simulink model "Galvo_sys_Cdisc_Pcont_cc_v64_proto_v13"  (R2013a)
settings: Solver=ode45  StartTime=0.0  StopTime=25e-3  FixedStep=FS  MaxStep=1e-5  RelTol=1e-3  AbsTol=1e-5
PreLoadFcn:
  | vname=@(x) inputname(1);
  | paramCtrl=evalin('base','paramCtrl;');
  | I_LIM=str2num(paramCtrl.I_LIM);
  | Kbc=str2num(paramCtrl.Kbc);
  | FS=evalin('base','FS;');
InitFcn:
  | %%%%%%  set scope time range
  | T_STOP=str2num(get_param(gcs,'StopTime'));
  | if numel(T_STOP) > 1
  |    T_STOP=T_STOP(2);
  | else
  |    T_STOP=T_STOP(1);
  | end
  | T_STOP=num2str(T_STOP);
  | 
  | %%%%%%  set scope time range in system @init_callback_fct
  | T_STOP=num2str(str2num(get_param(gcs,'StopTime')));
  | 
  | childs = allchild(0);
  | sol=strfind(upper(get(allchild(0),'Tag')),'VIEWER_PARAMETERS');
  | 
  | if iscell(sol)
  |    ind=find(~cellfun(@isempty, strfind(upper(get(allchild(0),'Tag')),'VIEWER_PARAMETERS')));
  | else
  |    ind=sol;
  | end
  | %ind=find(~cellfun(@isempty, {strfind(upper(get(allchild(0),'Tag')),'VIEWER_PARAMETERS'),[]}))
  | if ~isempty(ind)
  |    for k=1:length(childs(ind))
  |       set_param(getfield(get(childs(ind(k)),'UserData'),'block'),'TimeRange',T_STOP);
  |       get_param(getfield(get(childs(ind(k)),'UserData'),'block'),'TimeRange');
  | %    set_param(getfield(get(childs(ind),'UserData'),'block'),'TimeRange',T_STOP);
  | %    get_param(getfield(get(childs(ind),'UserData'),'block'),'TimeRange');
  |    end
  | else
  |     warning(sprintf('VIEWER_PARAMETERS object not found\nOpen the config dialog by hand for the first sim start'))
  | end
StartFcn:
  | I_LIM=str2num(paramCtrl.I_LIM);
  | Kbc=str2num(paramCtrl.Kbc);
  | %FS=evalin('base','FS;');
values from neighbouring files (symbols this model uses):
  Lc = 170e-6    (= 0.00017)    [GalvoModel_v6_sys.m]    (also in Galvo_process_analyze.m)
  Rc = 1.5    [GalvoModel_v6_sys.m]    (also in Galvo_process_analyze.m; frequenzgang_nichtinvert_opamp_koblitz_eas.m = 1)
  Rsh = 0.003    [GalvoModel_v6_sys.m]    (also in Galvo_sys_proto_v13_OFFSETS_MODEL_PT1B_proc.m = 0.075; frequenzgang_nichtinvert_opamp_koblitz_eas.m = 0.015)
undefined symbols (not defined in the file or in its folder): JR, KBM, KFR, KMT, KPOS1, KshM, KTB
libraries: simulink x4, simulink_extras x1, dspsigops x1
settings Model: BufferReuse=off  Creator=mainster  LastModifiedBy=mainster
settings SolverCC: AutoInsertRateTranBlk=on
settings DataIOCC: LimitDataPoints=off  SaveOutput=off  SaveTime=off
settings OptimizationCC: BlockReduction=off  InlineParams=on  OptimizeBlockIOStorage=off  BufferReuse=off  ExpressionFolding=off  LocalBlockOutputs=off
settings DebuggingCC: ArtificialAlgebraicLoopMsg=none  InitInArrayFormatMsg=none
settings HardwareCC: ProdLargestAtomicInteger=Long  ProdLargestAtomicFloat=Double  ProdEndianess=LittleEndian  ProdHWDeviceType=ARM Compatible->ARM Cortex
settings ModelReferenceCC: ModelReferenceNumInstancesAllowed=Single

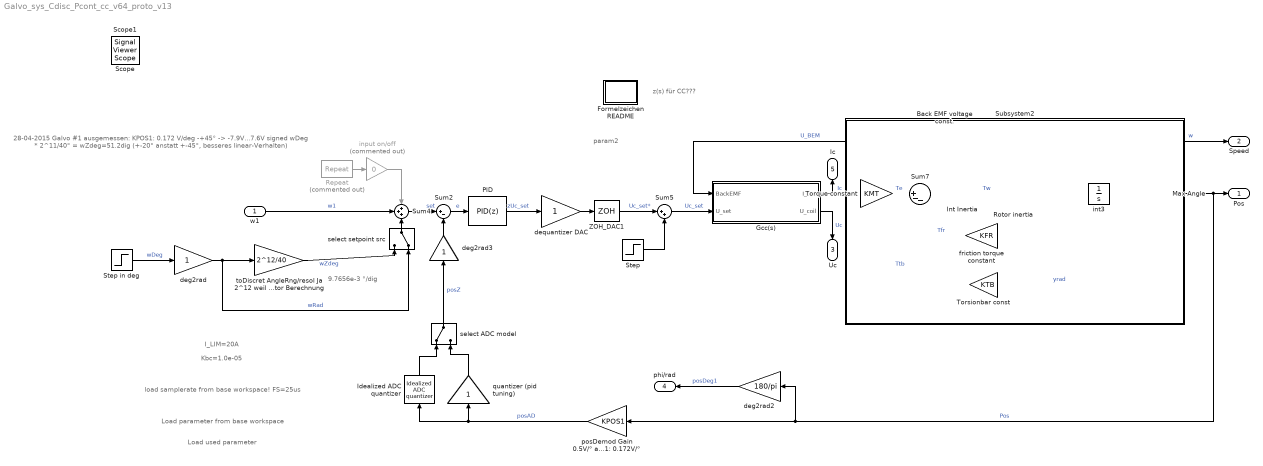
== system Galvo_sys_Cdisc_Pcont_cc_v64_proto_v13 ==
  note: 9.7656e-3 °/dig
  note: 28-04-2015
      | Galvo #1 ausgemessen:
      |
      | KPOS1: 0.172 V/deg
      |  -+45° ->  -7.9V...7.6V
      |
      | signed wDeg * 2^11/40° = wZdeg=51.2dig
      | (+-20° anstatt +-45°, besseres
      | linear-Verhalten)
  note: z(s) für
      | CC???
  note: param2
  note: I_LIM=20A
  note: Kbc=1.0e-05
  note: load samplerate from
      | base workspace!
      | FS=25us
  note: Load parameter from
      | base workspace
  note: Load used parameter
  w1 : Inport
  Back EMF voltage const. : Gain  Gain=KBM
  Formelzeichen README : Subsystem
  Gcc(s) : Subsystem
      mask Display:
      | %str=sprintf('%s',get(gcbh,'ModelName'));
      | port_label('input', 2, 'I/U_{Set}','texmode','on')
      | color('red');
      | port_label('input', 1, 'U_{BEM}','texmode','on')
      | color('black');
      | port_label('output', 1, 'I_{Coil}','texmode','on')
      | port_label('output', 2, 'U_{Coil}','texmode','on')
      | %text(.05,.98,['{\fontsize{12}\it\bf' strrep(str,'_',' ') '}'],'horizontalAlignment','left','verticalAlignment','top','texmode','on')
      | text(.5,0.95,['{\fontsize{12}\it\bfG_{cc}(s)}'],'horizontalAlignment','center','verticalAlignment','top','texmode','on')
      | %text(.5,0.45,['{\fontsize{8}\itKpcc=' num2str(get_param([gcb '/Cc(s)'],'P')) '}'],'horizontalAlignment','center','verticalAlignment','top','texmode','on')
      | %text(.5,0.25,['{\fontsize{8}\itKshM=' num2str(evalin('base',get_param([gcb '/shuntMonGain'],'Gain'))) '}'],'horizontalAlignment','center','verticalAlignment','top','texmode','on')
      | 
      | %text(.15,.05,['{\fontsize{10}\itmechanics}'],'horizontalAlignment','left','verticalAlignment','bottom','texmode','on')
  Idealized ADC quantizer : simulink_extras/Additional Discrete/Idealized ADC quantizer  NumberOfConverterBits=12  Vmin=-1.25  Vmax=1.25  OutputDataType=int16  OutputNegativeValues=on
  Int Inertia : Integrator
  Max Angle : Saturate  UpperLimit=20*pi/180*1e3  LowerLimit=-20*pi/180*1e3
      settings: AttributesFormatString=Max=%<UpperLimit>\nMin=%<LowerLimit>
  PID : simulink/Continuous/PID Controller  Controller=PID  TimeDomain=Discrete-time  SampleTime=FS  IntegratorMethod=Forward Euler  FilterMethod=Forward Euler  Form=Parallel  P=133.868463594608  I=12873.0781764522  D=0.158359314809688  N=29290.0509767599  InitialConditionSource=internal  InitialConditionForIntegrator=0  InitialConditionForFilter=0  ExternalReset=none  IgnoreLimit=on  LimitOutput=on  UpperSaturationLimit=2047  LowerSaturationLimit=-2048  LinearizeAsGain=off  AntiWindupMode=clamping  Kb=0.1  TrackingMode=off  Kt=0  PParamMin=[]  PParamMax=[]  IParamMin=[]  IParamMax=[]  DParamMin=[]  DParamMax=[]  NParamMin=[]  NParamMax=[]  KbParamMin=[]  KbParamMax=[]  KtParamMin=[]  KtParamMax=[]  POutMin=[]  POutMax=[]  IOutMin=[]  IOutMax=[]  DOutMin=[]  DOutMax=[]  NOutMin=[]  NOutMax=[]  KbOutMin=[]  KbOutMax=[]  KtOutMin=[]  KtOutMax=[]  IntegratorOutMin=[]  IntegratorOutMax=[]  FilterOutMin=[]  FilterOutMax=[]  SumOutMin=[]  SumOutMax=[]  SumI1OutMin=[]  SumI1OutMax=[]  SumI2OutMin=[]  SumI2OutMax=[]  SumI3OutMin=[]  SumI3OutMax=[]  SumDOutMin=[]  SumDOutMax=[]  SaturationOutMin=[]  SaturationOutMax=[]  IntegratorContinuousStateAttributes=''  IntegratorStateMustResolveToSignalObject=off  IntegratorRTWStateStorageClass=Auto  FilterContinuousStateAttributes=''  FilterStateMustResolveToSignalObject=off  FilterRTWStateStorageClass=Auto
      settings: AttributesFormatString=Kp: %<P>\nKi: %<I>\nKd: %<D>\nuplim: %<UpperSaturationLimit>\nlolim: %<LowerSaturationLimit>
  Repeat : dspsigops/Repeat  Commented=on  N=length(str2num(get_param([gcs '/Sequence Stair'], 'OutValues')))  InputProcessing=Columns as channels (frame based)  RateOptions=Allow multirate processing  ic=0  mode=Unused parameter value
  Rotor inertia : Gain  Gain=1/JR
  Step : Step  Time=100e-3  After=0  SampleTime=0
      settings: AttributesFormatString=Ampl.: %<After>\ntime:%<Time>
  Step in deg : Step  Time=1e-3  SampleTime=0  ZeroCross=off
      settings: AttributesFormatString=Ampl.: %<After>\ntime:%<Time>
  Subsystem2 : Subsystem
      mask Display: text(.05,.05,['{\fontsize{13}\it\bfGalvo mechanic}'],'horizontalAlignment','left','verticalAlignment','bottom','texmode','on')
  Sum2 : Sum  Inputs=|+-
  Sum4 : Sum  Inputs=+++
  Sum5 : Sum  Inputs=|++
  Sum7 : Sum  Inputs=||+--
  Torque constant : Gain  Gain=KMT
  Torsionbar const : Gain  Gain=KTB
  ZOH_DAC1 : ZeroOrderHold  SampleTime=FS
  deg2rad : Gain
  deg2rad2 : Gain  Gain=180/pi
  deg2rad3 : Gain
  dequantizer DAC : Gain
  friction torque constant : Gain  Gain=KFR
  input on/off : Gain  Commented=on  Gain=0  SampleTime=FS
  int3 : Integrator
  "posDemod Gain 0.5V/° ausgemessen bei Galvo #1: 0.172V/° " : Gain  Gain=KPOS1
  quantizer (pid tuning) : Gain
  select ADC model : ManualSwitch
  select setpoint src : ManualSwitch  CurrentSetting=0
  "toDiscret AngleRng/resol Ja 2^12 weil nur Faktor Berechnung " : Gain  Gain=2^12/40
  Pos : Outport
  Speed : Outport  Port=2
  Uc : Outport  Port=3
  phi/rad : Outport  Port=4
  Ic : Outport  Port=5
  Scope : SignalViewerScope  IOType=viewer  NumInputPorts=5  RefreshTime=0.033391
      settings: ShowLegends=on  TimeRange=0.025  YMin=0~-500~0~0~-500  YMax=8~2500~8~400~2500
  Scope1 : SignalViewerScope  IOType=viewer  NumInputPorts=5  RefreshTime=0.035000
      settings: ShowLegends=on  TimeRange=0.025  YMin=-10~0~-0.5~-20~0  YMax=10~1.5~1~30~120
  wires:
  w1/1 -> Sum4/2  "w1"
  Repeat/1 -> input on/off/1
  Sum2/1 -> PID/1  "e"
  Sum4/1 -> Sum2/1  "set"
  Step in deg/1 -> deg2rad/1  "wDeg"
  input on/off/1 -> Sum4/1
  Step/1 -> Sum5/2
  int3/1 -> Max Angle/1, Torsionbar const/1  "yrad"
  Int Inertia/1 -> Rotor inertia/1  "Tw"
  Sum7/1 -> Int Inertia/1
  Rotor inertia/1 -> Speed/1, int3/1, Back EMF voltage const./1, friction torque constant/1  "w"
  friction torque constant/1 -> Sum7/3  "Tfr"
  Max Angle/1 -> deg2rad2/1, "posDemod Gain 0.5V/° ausgemessen bei Galvo #1: 0.172V/° "/1, Pos/1  "Pos"
  Torque constant/1 -> Sum7/1  "Te"
  Torsionbar const/1 -> Sum7/2  "Ttb"
  PID/1 -> dequantizer DAC/1  "zUc_set"
  Sum5/1 -> Gcc(s)/2(U_set)  "Uc_set"
  Gcc(s)/1(I_coil) -> Torque constant/1, Ic/1  "Ic"
  Gcc(s)/2(U_coil) -> Uc/1  "Uc"
  "posDemod Gain 0.5V/° ausgemessen bei Galvo #1: 0.172V/° "/1 -> Idealized ADC quantizer/1, quantizer (pid tuning)/1  "posAD"
  deg2rad2/1 -> phi/rad/1  "posDeg1"
  Back EMF voltage const./1 -> Gcc(s)/1(BackEMF)  "U_BEM"
  ZOH_DAC1/1 -> Sum5/1  "Uc_set*"
  Idealized ADC quantizer/1 -> select ADC model/1
  select ADC model/1 -> deg2rad3/1  "posZ"
  "toDiscret AngleRng/resol Ja 2^12 weil nur Faktor Berechnung "/1 -> select setpoint src/1  "wZdeg"
  select setpoint src/1 -> Sum4/3
  deg2rad3/1 -> Sum2/2
  deg2rad/1 -> select setpoint src/2, "toDiscret AngleRng/resol Ja 2^12 weil nur Faktor Berechnung "/1  "wRad"
  quantizer (pid tuning)/1 -> select ADC model/2
  dequantizer DAC/1 -> ZOH_DAC1/1

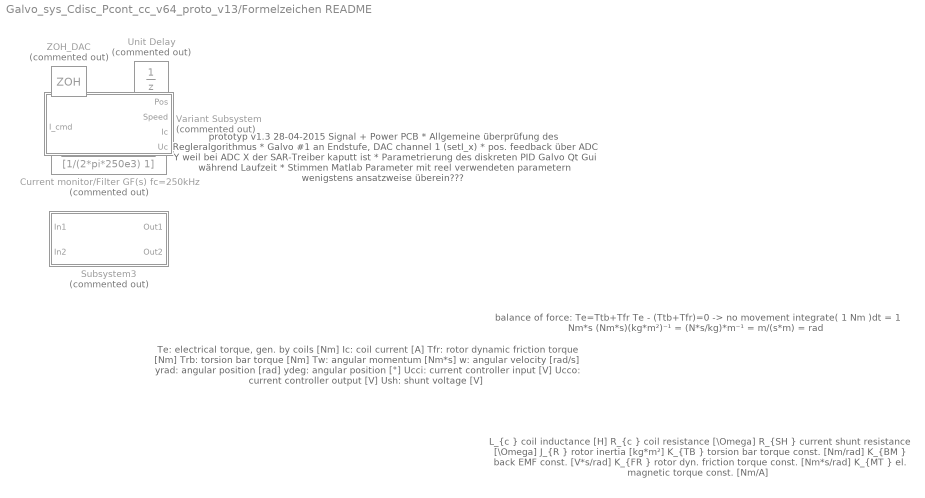
== system Galvo_sys_Cdisc_Pcont_cc_v64_proto_v13/Formelzeichen README ==
  note: Te: 		electrical torque, gen. by coils		[Nm]
      |  Ic: 			coil current							[A]
      |  Tfr:		rotor dynamic friction torque 		[Nm]
      |  Trb:		torsion bar torque					[Nm]
      |  Tw:		angular momentum				[Nm*s]
      |  w:			angular velocity 					[rad/s]
      |  yrad:		angular position 					[rad]
      |  ydeg:		angular position 					[°]
      |  Ucci:		current controller input				[V]
      |  Ucco:		current controller output			[V]
      |  Ush:		shunt voltage						[V]
  note: L_{c  }	coil inductance 							[H]
      |  R_{c  }	coil resistance							[\Omega]
      |  R_{SH }	current shunt resistance				[\Omega]
      |  J_{R  }	rotor inertia 							[kg*m²]
      |  K_{TB }	torsion bar torque const. 			[Nm/rad]
      |  K_{BM }	back EMF const.							[V*s/rad]
      |  K_{FR }	rotor dyn. friction torque const.	[Nm*s/rad]
      |  K_{MT }	el. magnetic torque const.			[Nm/A]
  note: balance of force: 	Te=Ttb+Tfr
      | 					Te - (Ttb+Tfr)=0  ->  no movement
      |
      |  integrate( 1 Nm )dt = 1 Nm*s
      |  (Nm*s)(kg*m²)⁻¹ = (N*s/kg)*m⁻¹ = m/(s*m) = rad
  note: prototyp v1.3
      | 28-04-2015
      |
      | Signal + Power PCB
      | * Allgemeine überprüfung des Regleralgorithmus
      | * Galvo #1 an Endstufe, DAC channel 1 (setI_x)
      | * pos. feedback über ADC Y weil bei ADC X der SAR-Treiber kaputt ist
      | * Parametrierung des diskreten PID Galvo Qt Gui während Laufzeit
      |
      | * Stimmen Matlab Parameter mit reel verwendeten parametern
      |   wenigstens ansatzweise überein???
  Current monitor/Filter GF(s) fc=250kHz : TransferFcn  Commented=on  Denominator=[1/(2*pi*250e3) 1]
  Subsystem3 : Subsystem  Commented=on
  Unit Delay : UnitDelay  Commented=on  SampleTime=-1
  Variant Subsystem : Subsystem  Commented=on  Variant=on  OverrideUsingVariant=Gv_CCsep
  ZOH_DAC : ZeroOrderHold  Commented=on

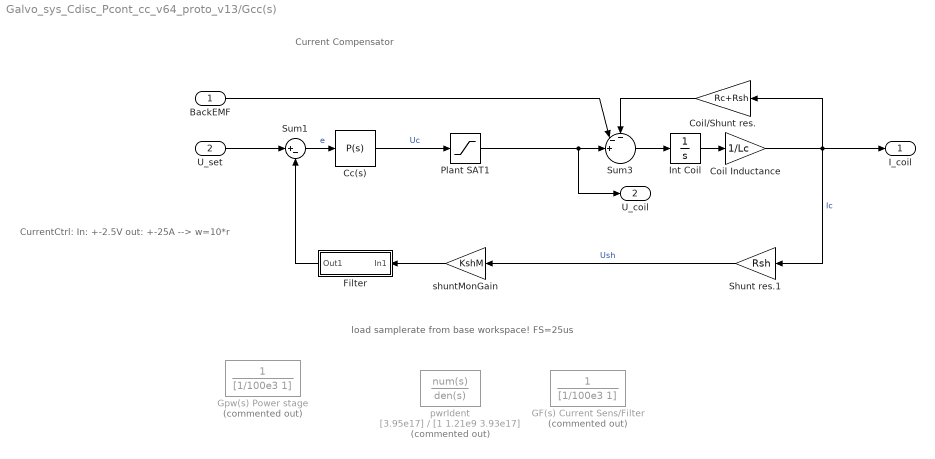
== system Galvo_sys_Cdisc_Pcont_cc_v64_proto_v13/Gcc(s) ==
  note: load samplerate from
      | base workspace!
      | FS=25us
  note: Current Compensator
  note: CurrentCtrl:
      | In:		+-2.5V
      | out: 	+-25A
      | --> w=10*r
  BackEMF : Inport
  U_set : Inport  Port=2
  Cc(s) : simulink/Continuous/PID Controller  Controller=P  TimeDomain=Continuous-time  SampleTime=-1  IntegratorMethod=Forward Euler  FilterMethod=Forward Euler  Form=Ideal  P=7.73423350237374  I=14078.2261040339  D=0  N=100  InitialConditionSource=internal  InitialConditionForIntegrator=0  InitialConditionForFilter=0  ExternalReset=none  LimitOutput=off  UpperSaturationLimit=inf  LowerSaturationLimit=-inf  LinearizeAsGain=on  AntiWindupMode=none  Kb=1  TrackingMode=off  Kt=1  PParamMin=[]  PParamMax=[]  IParamMin=[]  IParamMax=[]  DParamMin=[]  DParamMax=[]  NParamMin=[]  NParamMax=[]  KbParamMin=[]  KbParamMax=[]  KtParamMin=[]  KtParamMax=[]  POutMin=[]  POutMax=[]  IOutMin=[]  IOutMax=[]  DOutMin=[]  DOutMax=[]  NOutMin=[]  NOutMax=[]  KbOutMin=[]  KbOutMax=[]  KtOutMin=[]  KtOutMax=[]  IntegratorOutMin=[]  IntegratorOutMax=[]  FilterOutMin=[]  FilterOutMax=[]  SumOutMin=[]  SumOutMax=[]  SumI1OutMin=[]  SumI1OutMax=[]  SumI2OutMin=[]  SumI2OutMax=[]  SumI3OutMin=[]  SumI3OutMax=[]  SumDOutMin=[]  SumDOutMax=[]  SaturationOutMin=[]  SaturationOutMax=[]  IntegratorContinuousStateAttributes=''  IntegratorStateMustResolveToSignalObject=off  IntegratorRTWStateStorageClass=Auto  FilterContinuousStateAttributes=''  FilterStateMustResolveToSignalObject=off  FilterRTWStateStorageClass=Auto
      settings: AttributesFormatString=Kp: %<P>\nuplim: %<UpperSaturationLimit>\nlolim: %<LowerSaturationLimit>
  Coil Inductance : Gain  Gain=1/Lc
  Coil/Shunt res. : Gain  Gain=Rc+Rsh
  Filter : Subsystem
  GF(s) Current Sens/Filter : TransferFcn  Commented=on  Denominator=[1/100e3 1]
  Gpw(s) Power stage : TransferFcn  Commented=on  Denominator=[1/100e3 1]
  Int Coil : Integrator
  Plant SAT1 : Saturate  UpperLimit=30  LowerLimit=-30
      settings: AttributesFormatString=U_lim=+-%<UpperLimit>V
  Shunt res.1 : Gain  Gain=Rsh
  Sum1 : Sum  Inputs=|+-
  Sum3 : Sum  Inputs=--+||
  pwrIdent : TransferFcn  Commented=on  Numerator=[3.95e17]  Denominator=[1 1.21e9 3.93e17]
  shuntMonGain : Gain  Gain=KshM
  I_coil : Outport
  U_coil : Outport  Port=2
  wires:
  Cc(s)/1 -> Plant SAT1/1  "Uc"
  BackEMF/1 -> Sum3/2
  Shunt res.1/1 -> shuntMonGain/1  "Ush"
  Plant SAT1/1 -> U_coil/1, Sum3/3
  Sum1/1 -> Cc(s)/1  "e"
  Coil Inductance/1 -> I_coil/1, Shunt res.1/1, Coil/Shunt res./1  "Ic"
  Coil/Shunt res./1 -> Sum3/1
  Sum3/1 -> Int Coil/1
  Int Coil/1 -> Coil Inductance/1
  U_set/1 -> Sum1/1
  shuntMonGain/1 -> Filter/1(In1)
  Filter/1(Out1) -> Sum1/2

== system Galvo_sys_Cdisc_Pcont_cc_v64_proto_v13/Subsystem2 ==

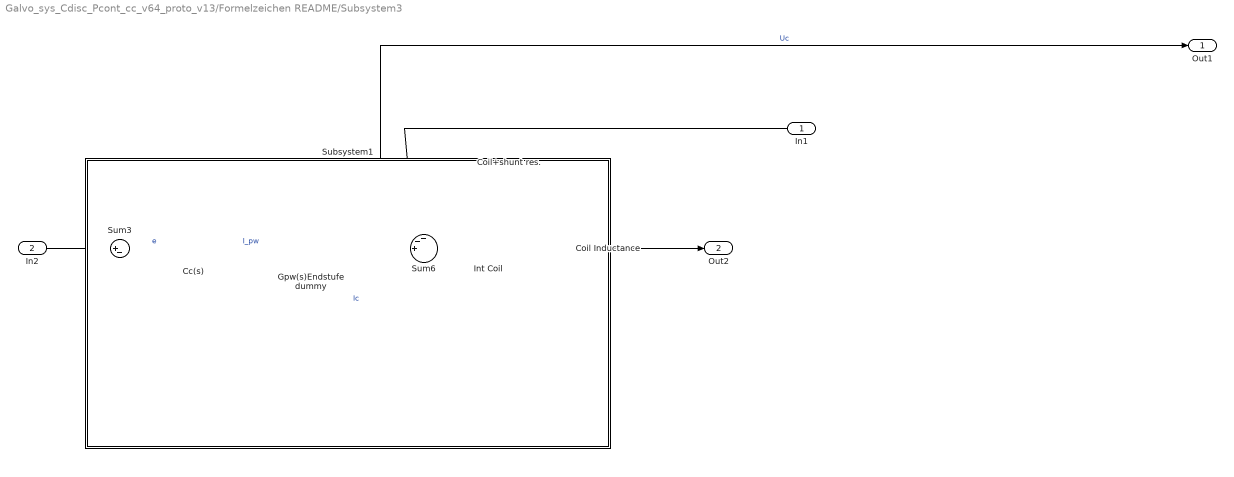
== system Galvo_sys_Cdisc_Pcont_cc_v64_proto_v13/Formelzeichen README/Subsystem3 ==
  In1 : Inport
  In2 : Inport  Port=2
  Cc(s) : simulink/Continuous/PID Controller  Controller=P  TimeDomain=Continuous-time  SampleTime=-1  IntegratorMethod=Forward Euler  FilterMethod=Forward Euler  Form=Ideal  P=59.6963088947406  I=1985.39023021624  D=0  N=100  InitialConditionSource=internal  InitialConditionForIntegrator=0  InitialConditionForFilter=0  ExternalReset=none  LimitOutput=off  UpperSaturationLimit=inf  LowerSaturationLimit=-inf  LinearizeAsGain=on  AntiWindupMode=none  Kb=1  TrackingMode=off  Kt=1  PParamMin=[]  PParamMax=[]  IParamMin=[]  IParamMax=[]  DParamMin=[]  DParamMax=[]  NParamMin=[]  NParamMax=[]  KbParamMin=[]  KbParamMax=[]  KtParamMin=[]  KtParamMax=[]  POutMin=[]  POutMax=[]  IOutMin=[]  IOutMax=[]  DOutMin=[]  DOutMax=[]  NOutMin=[]  NOutMax=[]  KbOutMin=[]  KbOutMax=[]  KtOutMin=[]  KtOutMax=[]  IntegratorOutMin=[]  IntegratorOutMax=[]  FilterOutMin=[]  FilterOutMax=[]  SumOutMin=[]  SumOutMax=[]  SumI1OutMin=[]  SumI1OutMax=[]  SumI2OutMin=[]  SumI2OutMax=[]  SumI3OutMin=[]  SumI3OutMax=[]  SumDOutMin=[]  SumDOutMax=[]  SaturationOutMin=[]  SaturationOutMax=[]  IntegratorContinuousStateAttributes=''  IntegratorStateMustResolveToSignalObject=off  IntegratorRTWStateStorageClass=Auto  FilterContinuousStateAttributes=''  FilterStateMustResolveToSignalObject=off  FilterRTWStateStorageClass=Auto
      settings: AttributesFormatString=P = %<P>
  Coil Inductance : Gain  Gain=1/Lc
  Coil+shunt res. : Gain  Gain=Rc+Rsh
  Gpw(s)Endstufe dummy : Gain
  Int Coil : Integrator
  Subsystem1 : Subsystem
      mask Display: text(.05,.90,['{\fontsize{13}\it\bfCurrent Compensator}'],'horizontalAlignment','left','verticalAlignment','bottom','texmode','on')
  Sum3 : Sum  Inputs=|+-
  Sum6 : Sum  Inputs=--+||
  Out1 : Outport
  Out2 : Outport  Port=2
  wires:
  Int Coil/1 -> Coil Inductance/1
  Coil Inductance/1 -> Out2/1, Sum3/2, Coil+shunt res./1  "Ic"
  Coil+shunt res./1 -> Sum6/1
  Gpw(s)Endstufe dummy/1 -> Out1/1, Sum6/3  "Uc"
  In2/1 -> Sum3/1
  Sum6/1 -> Int Coil/1
  Sum3/1 -> Cc(s)/1  "e"
  Cc(s)/1 -> Gpw(s)Endstufe dummy/1  "I_pw"
  In1/1 -> Sum6/2

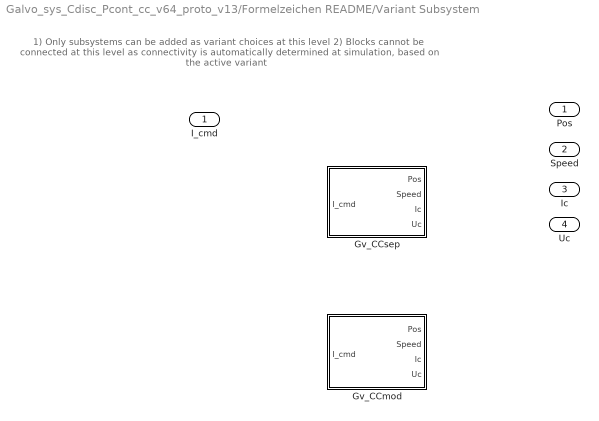
== system Galvo_sys_Cdisc_Pcont_cc_v64_proto_v13/Formelzeichen README/Variant Subsystem ==
  note: 1) Only subsystems can be added as variant choices at this level
      | 2) Blocks cannot be connected at this level as connectivity is
      | automatically determined at simulation, based on the active variant
  I_cmd : Inport
  Gv_CCmod : Subsystem  VariantControl=Gv_CCmod
  Gv_CCsep : Subsystem  VariantControl=Gv_CCsep
  Pos : Outport  SampleTime=FS
  Speed : Outport  Port=2  SampleTime=FS
  Ic : Outport  Port=3  SampleTime=FS
  Uc : Outport  Port=4  SampleTime=FS

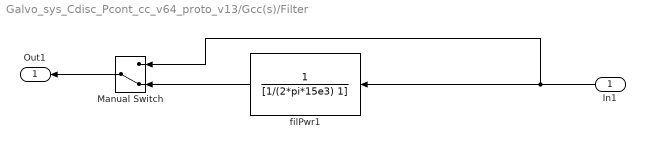
== system Galvo_sys_Cdisc_Pcont_cc_v64_proto_v13/Gcc(s)/Filter ==
  In1 : Inport
  Manual Switch : ManualSwitch  CurrentSetting=0
  filPwr1 : TransferFcn  Denominator=[1/(2*pi*15e3) 1]
  Out1 : Outport
  wires:
  Manual Switch/1 -> Out1/1
  filPwr1/1 -> Manual Switch/2
  In1/1 -> filPwr1/1, Manual Switch/1

== system Galvo_sys_Cdisc_Pcont_cc_v64_proto_v13/Formelzeichen README/Subsystem3/Subsystem1 ==

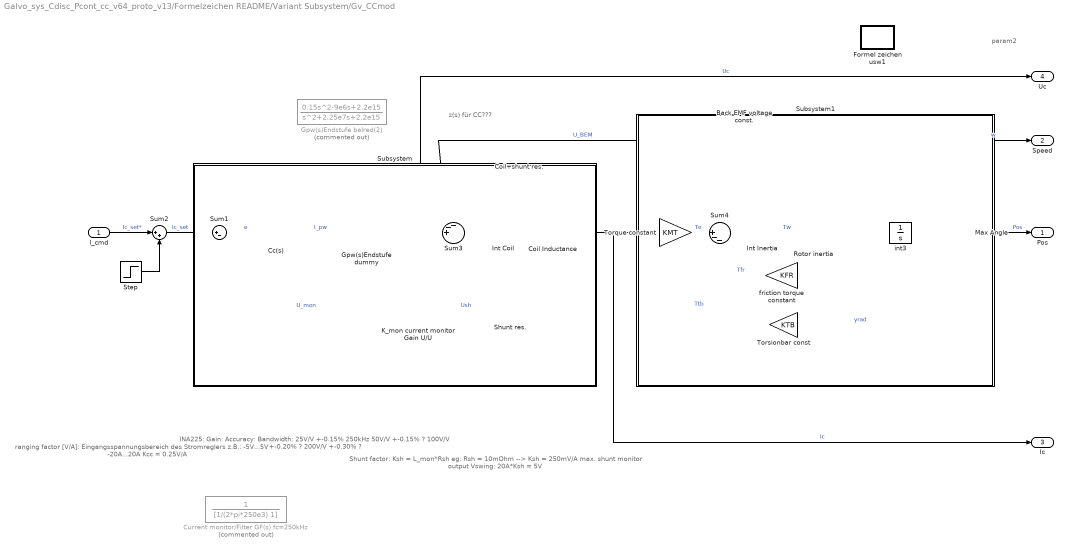
== system Galvo_sys_Cdisc_Pcont_cc_v64_proto_v13/Formelzeichen README/Variant Subsystem/Gv_CCmod ==
  note: z(s) für
      | CC???
  note: ranging factor [V/A]:
      | Eingangsspannungsbereich des
      | Stromreglers z.B.:
      | -5V...5V --> -20A...20A
      | Kcc = 0.25V/A
  note: Shunt factor:
      | Ksh = L_mon*Rsh
      |
      | eg: Rsh = 10mOhm
      |
      | --> Ksh = 250mV/A
      | max. shunt monitor
      | output Vswing:
      | 20A*Ksh = 5V
  note: INA225:
      | Gain:		Accuracy:		Bandwidth:
      | 25V/V		+-0.15%		250kHz
      | 50V/V		+-0.15%		?
      | 100V/V	+-0.20%		?
      | 200V/V	+-0.30%		?
  note: param2
  I_cmd : Inport  SampleTime=FS
  Back EMF voltage const. : Gain  Gain=KBM
  Cc(s) : simulink/Continuous/PID Controller  Controller=P  TimeDomain=Continuous-time  SampleTime=-1  IntegratorMethod=Forward Euler  FilterMethod=Forward Euler  Form=Ideal  P=15.5227390982487  I=1985.39023021624  D=0  N=100  InitialConditionSource=internal  InitialConditionForIntegrator=0  InitialConditionForFilter=0  ExternalReset=none  LimitOutput=off  UpperSaturationLimit=inf  LowerSaturationLimit=-inf  LinearizeAsGain=on  AntiWindupMode=none  Kb=1  TrackingMode=off  Kt=1  PParamMin=[]  PParamMax=[]  IParamMin=[]  IParamMax=[]  DParamMin=[]  DParamMax=[]  NParamMin=[]  NParamMax=[]  KbParamMin=[]  KbParamMax=[]  KtParamMin=[]  KtParamMax=[]  POutMin=[]  POutMax=[]  IOutMin=[]  IOutMax=[]  DOutMin=[]  DOutMax=[]  NOutMin=[]  NOutMax=[]  KbOutMin=[]  KbOutMax=[]  KtOutMin=[]  KtOutMax=[]  IntegratorOutMin=[]  IntegratorOutMax=[]  FilterOutMin=[]  FilterOutMax=[]  SumOutMin=[]  SumOutMax=[]  SumI1OutMin=[]  SumI1OutMax=[]  SumI2OutMin=[]  SumI2OutMax=[]  SumI3OutMin=[]  SumI3OutMax=[]  SumDOutMin=[]  SumDOutMax=[]  SaturationOutMin=[]  SaturationOutMax=[]  IntegratorContinuousStateAttributes=''  IntegratorStateMustResolveToSignalObject=off  IntegratorRTWStateStorageClass=Auto  FilterContinuousStateAttributes=''  FilterStateMustResolveToSignalObject=off  FilterRTWStateStorageClass=Auto
      settings: AttributesFormatString=P = %<P>
  Coil Inductance : Gain  Gain=1/Lc
  Coil+shunt res. : Gain  Gain=Rc+Rsh
  Current monitor/Filter GF(s) fc=250kHz : TransferFcn  Commented=on  Denominator=[1/(2*pi*250e3) 1]
  Formel zeichen usw1 : Subsystem
  Gpw(s)Endstufe balred(2) : TransferFcn  Commented=on  Numerator=[0.15 -9e6 2.2e15]  Denominator=[1 2.25e7 2.2e15]
  Gpw(s)Endstufe dummy : Gain
  Int Coil : Integrator
  Int Inertia : Integrator
  K_mon current monitor Gain U/U : Gain  Gain=1/Rsh
  Max Angle : Saturate  UpperLimit=20*pi/180  LowerLimit=-20*pi/180
      settings: AttributesFormatString=Max=%<UpperLimit>\nMin=%<LowerLimit>
  Rotor inertia : Gain  Gain=1/JR
  Shunt res. : Gain  Gain=Rsh
  Step : Step  Time=0
      settings: AttributesFormatString=%<Time>
  Subsystem : Subsystem
      mask Display: text(.05,.90,['{\fontsize{13}\it\bfCurrent Compensator}'],'horizontalAlignment','left','verticalAlignment','bottom','texmode','on')
  Subsystem1 : Subsystem
      mask Display: text(.05,.05,['{\fontsize{13}\it\bfGalvo mechanic}'],'horizontalAlignment','left','verticalAlignment','bottom','texmode','on')
  Sum1 : Sum  Inputs=|+-
  Sum2 : Sum  Inputs=|++
  Sum3 : Sum  Inputs=--+||
  Sum4 : Sum  Inputs=||+--
  Torque constant : Gain  Gain=KMT
  Torsionbar const : Gain  Gain=KTB
  friction torque constant : Gain  Gain=KFR
  int3 : Integrator
  Pos : Outport  SampleTime=FS
  Speed : Outport  Port=2  SampleTime=FS
  Ic : Outport  Port=3  SampleTime=FS
  Uc : Outport  Port=4  SampleTime=FS
  wires:
  I_cmd/1 -> Sum2/1  "Ic_set*"
  Sum1/1 -> Cc(s)/1  "e"
  Sum3/1 -> Int Coil/1
  Int Coil/1 -> Coil Inductance/1
  Cc(s)/1 -> Gpw(s)Endstufe dummy/1  "I_pw"
  K_mon current monitor Gain U/U/1 -> Sum1/2  "U_mon"
  Shunt res./1 -> K_mon current monitor Gain U/U/1  "Ush"
  Gpw(s)Endstufe dummy/1 -> Uc/1, Sum3/3  "Uc"
  Coil+shunt res./1 -> Sum3/1
  Sum2/1 -> Sum1/1  "Ic_set"
  Step/1 -> Sum2/2
  int3/1 -> Max Angle/1, Torsionbar const/1  "yrad"
  Int Inertia/1 -> Rotor inertia/1  "Tw"
  Sum4/1 -> Int Inertia/1
  Rotor inertia/1 -> Speed/1, int3/1, Back EMF voltage const./1, friction torque constant/1  "w"
  friction torque constant/1 -> Sum4/3  "Tfr"
  Max Angle/1 -> Pos/1  "Pos"
  Coil Inductance/1 -> Ic/1, Torque constant/1, Coil+shunt res./1, Shunt res./1  "Ic"
  Back EMF voltage const./1 -> Sum3/2  "U_BEM"
  Torque constant/1 -> Sum4/1  "Te"
  Torsionbar const/1 -> Sum4/2  "Ttb"

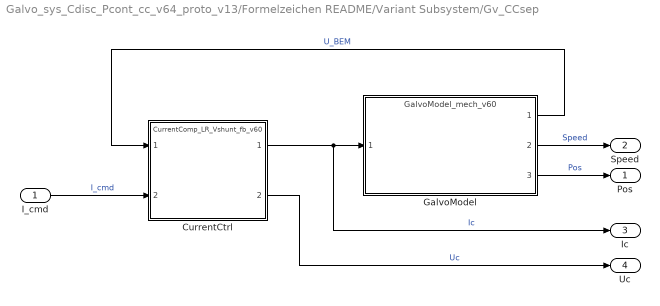
== system Galvo_sys_Cdisc_Pcont_cc_v64_proto_v13/Formelzeichen README/Variant Subsystem/Gv_CCsep ==
  I_cmd : Inport  SampleTime=FS
  CurrentCtrl : ModelReference  ModelNameDialog=CurrentComp_LR_Vshunt_fb_v60.slx  SimulationMode=Normal  Variant=on  OverrideUsingVariant=cc_v20  ModelReferenceVersion=1.94  CopyOfModelName=CurrentComp_LR_Vshunt_fb_v60.slx  DefaultDataLogging=on
      mask Display:
      | str=sprintf('%s',get(gcbh,'ModelName'));
      | port_label('input', 2, 'I_{Set}','texmode','on')
      | color('red');
      | port_label('input', 1, 'U_{BEM}','texmode','on')
      | color('black');
      | port_label('output', 1, 'I_{Coil}','texmode','on')
      | port_label('output', 2, 'U_{Coil}','texmode','on')
      | %text(.05,.98,['{\fontsize{12}\it\bf' strrep(str,'_',' ') '}'],'horizontalAlignment','left','verticalAlignment','top','texmode','on')
      | text(.5,0.95,['{\fontsize{12}\it\bfG_{cc}(s)}'],'horizontalAlignment','center','verticalAlignment','top','texmode','on')
      | %text(.15,.05,['{\fontsize{10}\itmechanics}'],'horizontalAlignment','left','verticalAlignment','bottom','texmode','on')
  GalvoModel : ModelReference  ModelNameDialog=GalvoModel_mech_v60.slx  SimulationMode=Normal  Variant=on  OverrideUsingVariant=v53_neuer_cc  ModelReferenceVersion=1.68  CopyOfModelName=GalvoModel_mech_v60.slx  DefaultDataLogging=on
      mask Display:
      | str=sprintf('%s',get(gcbh,'ModelName'));
      | port_label('input', 1, 'I_{Coil}','texmode','on')
      | color('blue');
      | port_label('output', 3, 'Pos','texmode','on')
      | color('black');
      | port_label('output', 2, 'Speed','texmode','on')
      | port_label('output', 1, 'U_{BEM}','texmode','on')
      | %text(.05,.98,['{\fontsize{12}\it\bf' strrep(str,'_',' ') '}'],'horizontalAlignment','left','verticalAlignment','top','texmode','on')
      | text(.015,.98,['{\fontsize{12}\it\bf' strrep(str,'_','\_') '}'],'horizontalAlignment','left','verticalAlignment','top','texmode','on')
      | text(.15,.05,['{\fontsize{10}\itmechanics}'],'horizontalAlignment','left','verticalAlignment','bottom','texmode','on')
  Pos : Outport  SampleTime=FS
  Speed : Outport  Port=2  SampleTime=FS
  Ic : Outport  Port=3  SampleTime=FS
  Uc : Outport  Port=4  SampleTime=FS
  wires:
  CurrentCtrl/1 -> GalvoModel/1, Ic/1  "Ic"
  GalvoModel/2 -> Speed/1  "Speed"
  GalvoModel/3 -> Pos/1  "Pos"
  GalvoModel/1 -> CurrentCtrl/1  "U_BEM"
  I_cmd/1 -> CurrentCtrl/2  "I_cmd"
  CurrentCtrl/2 -> Uc/1  "Uc"

== system Galvo_sys_Cdisc_Pcont_cc_v64_proto_v13/Formelzeichen README/Variant Subsystem/Gv_CCmod/Formel zeichen usw1 ==
  note: Te: 		electrical torque, gen. by coils		[Nm]
      |  Ic: 			coil current							[A]
      |  Tfr:		rotor dynamic friction torque 		[Nm]
      |  Trb:		torsion bar torque					[Nm]
      |  Tw:		angular momentum				[Nm*s]
      |  w:			angular velocity 					[rad/s]
      |  yrad:		angular position 					[rad]
      |  ydeg:		angular position 					[°]
      |  Ucci:		current controller input				[V]
      |  Ucco:		current controller output			[V]
      |  Ush:		shunt voltage						[V]
  note: L_{c  }	coil inductance 							[H]
      |  R_{c  }	coil resistance							[\Omega]
      |  R_{SH }	current shunt resistance				[\Omega]
      |  J_{R  }	rotor inertia 							[kg*m²]
      |  K_{TB }	torsion bar torque const. 			[Nm/rad]
      |  K_{BM }	back EMF const.							[V*s/rad]
      |  K_{FR }	rotor dyn. friction torque const.	[Nm*s/rad]
      |  K_{MT }	el. magnetic torque const.			[Nm/A]
  note: balance of force: 	Te=Ttb+Tfr
      | 					Te - (Ttb+Tfr)=0  ->  no movement
      |
      |  integrate( 1 Nm )dt = 1 Nm*s
      |  (Nm*s)(kg*m²)⁻¹ = (N*s/kg)*m⁻¹ = m/(s*m) = rad

== system Galvo_sys_Cdisc_Pcont_cc_v64_proto_v13/Formelzeichen README/Variant Subsystem/Gv_CCmod/Subsystem ==

== system Galvo_sys_Cdisc_Pcont_cc_v64_proto_v13/Formelzeichen README/Variant Subsystem/Gv_CCmod/Subsystem1 ==
